simulink model "LongDyn2"  (R2017a)
settings: Solver=VariableStepAuto  StartTime=0.0  StopTime=10.0  RelTol=1e-3
undefined symbols (not defined in the file): sigbuilder_block
settings Model: Creator=Soutrik  LastModifiedBy=Soutrik

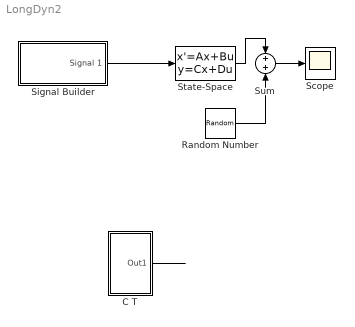
== system LongDyn2 ==
  C T : Subsystem
  Random Number : RandomNumber  Variance=[0.0001, 0.0000001, 0.00002, 0.00002]  SampleTime=0.01
  Scope : Scope
  Signal Builder : Subsystem  Tag=STV Subsys  LoadFcn=sigbuilder_block('load');  StartFcn=sigbuilder_block('start');  StopFcn=sigbuilder_block('stop');  ClipboardFcn=sigbuilder_block('clipboard');  mask(Sigbuilder block){tuvar=[0:10]}
      mask help: Simulink:masks:SigbuilderBlock_MD
      mask init:
      | if ~strcmp(get_param(bdroot(gcbh),'SimulationStatus'),'stopped') tuvar = sigbuilder_block('maskInit'); end
      settings: CopyFcn=sigbuilder_block('copy');  DeleteFcn=sigbuilder_block('delete');  ModelCloseFcn=sigbuilder_block('modelClose');  PreSaveFcn=sigbuilder_block('preSave');  PauseFcn=sigbuilder_block('pause');  ContinueFcn=sigbuilder_block('continue');  NameChangeFcn=sigbuilder_block('namechange');  OpenFcn=sigbuilder_block('open',[300 184.875 550.5 400.125 ]);  CloseFcn=sigbuilder_block('close');
      mask Display: plot(0, 0, 100, 100,[2, 2, 32, 32, 2], [68, 8, 8, 68, 68],[32, 2], [38, 38], [32, 19, 2],[53, 60, 44], [32, 17, 17, 2],[16, 16, 31, 31]);txt = getActiveGroup(gcbh);text(2, 100, txt,'verticalAlignment', 'top');
  State-Space : StateSpace  A=|  B=|  C=|  D=[0;0;0;0];  X0=0
      A=|
      | [0 1.0000 0 0;
      | 0 -0.9965 0 -0.3000;
      | -0.3197 -0.5176 -0.0100 -0.7000;
      | 0 0 -0.0005 -0.9924];
      B=|
      | [ 0;
      | -0.0013;
      | 0.0001;
      | -0.0201];
      C=|
      | [0 0 0.9963 0.0862;
      | 0 0 -0.0001 0.0017;
      | 1.0000 0 0 0;
      | 0 1.0000 0 0];
  Sum : Sum  Inputs=2
  wires:
  C T/1(Out1) -> ?
  Sum/1 -> Scope/1
  Random Number/1 -> Sum/2
  State-Space/1 -> Sum/1
  Signal Builder/1(Signal 1) -> State-Space/1

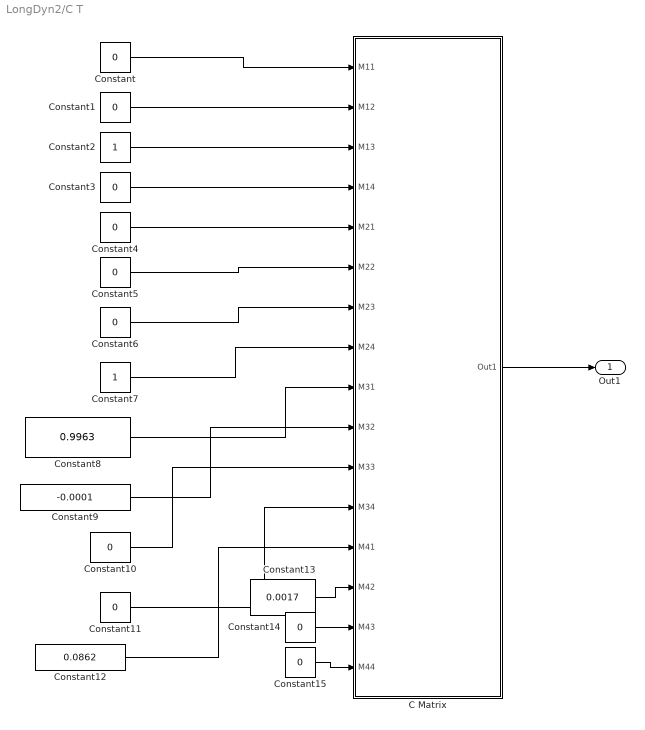
== system LongDyn2/C T ==
  C Matrix : Subsystem
  Constant{,1,3..6,10..11,14..15} (10 alike) : Constant  Value=0
  Constant12 : Constant  Value=0.0862
  Constant13 : Constant  Value=0.0017
  Constant2 : Constant
  Constant7 : Constant
  Constant8 : Constant  Value=0.9963
  Constant9 : Constant  Value=-0.0001
  Out1 : Outport
  wires:
  Constant1/1 -> C Matrix/2(M12)
  Constant13/1 -> C Matrix/14(M42)
  C Matrix/1(Out1) -> Out1/1
  Constant5/1 -> C Matrix/6(M22)
  Constant2/1 -> C Matrix/3(M13)
  Constant15/1 -> C Matrix/16(M44)
  Constant11/1 -> C Matrix/12(M34)
  Constant14/1 -> C Matrix/15(M43)
  Constant/1 -> C Matrix/1(M11)
  Constant12/1 -> C Matrix/13(M41)
  Constant7/1 -> C Matrix/8(M24)
  Constant10/1 -> C Matrix/11(M33)
  Constant4/1 -> C Matrix/5(M21)
  Constant3/1 -> C Matrix/4(M14)
  Constant8/1 -> C Matrix/9(M31)
  Constant6/1 -> C Matrix/7(M23)
  Constant9/1 -> C Matrix/10(M32)

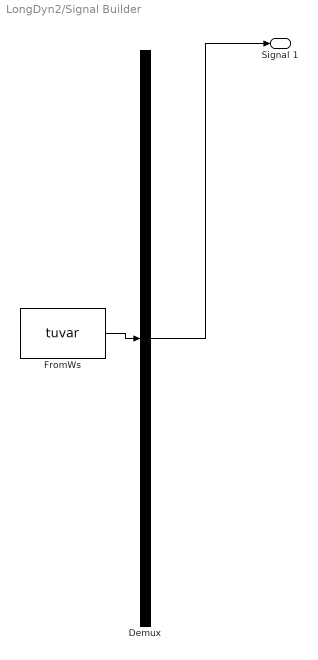
== system LongDyn2/Signal Builder ==
  Demux : Demux  Tag=STV Demux  Outputs=1
  FromWs : FromWorkspace  Tag=STV FromWs  VariableName=tuvar  SampleTime=0
      SigBuilderData=|
      | common.afterFinalStr = 'Extrapolate'
      | common.sampleTime = 0
      | dataSet.timeRange = [0 10]
      | dataSet.name = 'Group 1'
      | sbobj.Groups.Name = 'Group 1'
      | sbobj.Groups.Signals.Name = 'Signal 1'
      | sbobj.Groups.Signals.XData = [0 1.02 1.02 2.04 2.04 3.04 3.04 10]
      | sbobj.Groups.Signals.YData = [0 -0.002 50 50 -50 -50 0 0]
  Signal 1 : Outport  Tag=STV Outport
  wires:
  Demux/1 -> Signal 1/1
  FromWs/1 -> Demux/1

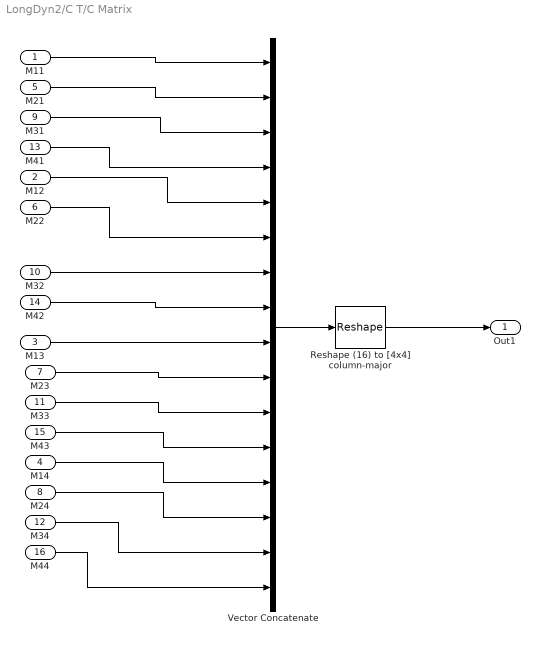
== system LongDyn2/C T/C Matrix ==
  M11 : Inport  PortDimensions=1
  M12 : Inport  Port=2  PortDimensions=1
  M13 : Inport  Port=3  PortDimensions=1
  M14 : Inport  Port=4  PortDimensions=1
  M21 : Inport  Port=5  PortDimensions=1
  M22 : Inport  Port=6  PortDimensions=1
  M23 : Inport  Port=7  PortDimensions=1
  M24 : Inport  Port=8  PortDimensions=1
  M31 : Inport  Port=9  PortDimensions=1
  M32 : Inport  Port=10  PortDimensions=1
  M33 : Inport  Port=11  PortDimensions=1
  M34 : Inport  Port=12  PortDimensions=1
  M41 : Inport  Port=13  PortDimensions=1
  M42 : Inport  Port=14  PortDimensions=1
  M43 : Inport  Port=15  PortDimensions=1
  M44 : Inport  Port=16  PortDimensions=1
  Reshape (16) to [4x4] column-major : Reshape  OutputDimensionality=Customize  OutputDimensions=[4,4]
  Vector Concatenate : Concatenate  NumInputs=16
  Out1 : Outport
  wires:
  M32/1 -> Vector Concatenate/7
  Vector Concatenate/1 -> Reshape (16) to [4x4] column-major/1
  Reshape (16) to [4x4] column-major/1 -> Out1/1
  M42/1 -> Vector Concatenate/8
  M22/1 -> Vector Concatenate/6
  M13/1 -> Vector Concatenate/9
  M21/1 -> Vector Concatenate/2
  M31/1 -> Vector Concatenate/3
  M11/1 -> Vector Concatenate/1
  M41/1 -> Vector Concatenate/4
  M12/1 -> Vector Concatenate/5
  M14/1 -> Vector Concatenate/13
  M33/1 -> Vector Concatenate/11
  M34/1 -> Vector Concatenate/15
  M44/1 -> Vector Concatenate/16
  M23/1 -> Vector Concatenate/10
  M43/1 -> Vector Concatenate/12
  M24/1 -> Vector Concatenate/14
